simulink model "Rectifier_Buck_Model_rev05_with_Termal_Power_Measurement"  (R2020b)
settings: Solver=VariableStepAuto  StartTime=0.0  StopTime=10  RelTol=1e-3
values from neighbouring files (symbols this model uses):
  L = Vout*(1-D)/(fs*delta_i)    (= 0.001104)    [Parameters.m]
undefined symbols (not defined in the file or in its folder): Acid, Lead
libraries: powerlib x18, electricdrivelib x1, powerlib_meascontrol x1
settings Model: Creator=Alper  LastModifiedBy=faati

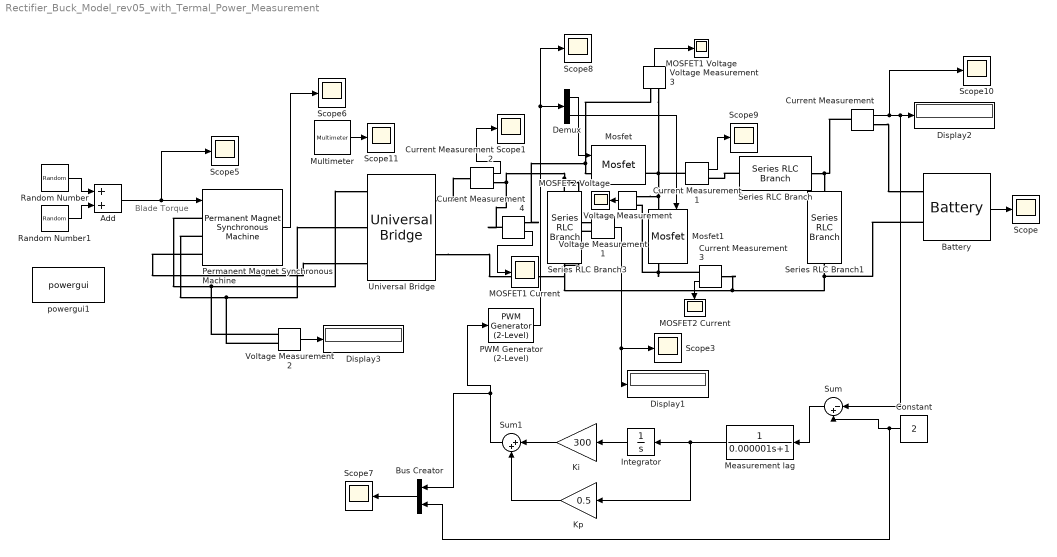
== system Rectifier_Buck_Model_rev05_with_Termal_Power_Measurement ==
  note: Blade Torque
  Add : Sum
  Battery : electricdrivelib/Extra Sources/Battery  BatType=Lead-Acid  ShowTempParam=off  ThermalPreset=no  ShowAgeParam=off  NomV=24  NomQ=5.4  SOC=50  Batt_Tr=30  PresetModel=off  MaxQ=5.625  MinV=18  FullV=26.1316  Dis_rate=1.08  R=0.044444  Normal_OP=1.6755  expZone="[24.4342        0.018]"  current=[6.5 13 32.5]  Units=Time  Tci=20  NomT=20  T2=-30  MaxQ2=4.8  FullV2=7.1  Normal_OP2=5.655  expZone2="[6.58           1]"  Rca=0.6  ti=2000  Dp=0  Neq0=0  Tsim=1e6  Ta1=25  Qeol=5.4*0.9  Reol=0.013333*1.2  Char_age=[2.3478, 3]  Dis_age=[2.3478, 10]  N1=1500  N2=10500  N3=1000  N4=1400  Ta2=45  N5=950
  Bus Creator : BusCreator  Inputs=2
  Constant : Constant  Value=2
  Current Measurement{,1..4} (5 alike) : powerlib/Measurements/Current Measurement  PhasorSimulation=off  OutputType=Complex  PSBequivalent=0
  Demux : Demux  Outputs=2
  Display1 : Display
  Display2 : Display
  Display3 : Display
  Integrator : Integrator
  Ki : Gain  Gain=300
  Kp : Gain  Gain=0.5
  MOSFET1 Current : Scope
  MOSFET1 Voltage : Scope
  MOSFET2 Current : Scope
  MOSFET2 Voltage : Scope
  Measurement lag : TransferFcn  Denominator=[0.000001 1]
  Mosfet : powerlib/Power Electronics/Mosfet  Ron=0.1  Lon=0  Rd=0.01  Vfd=0  IC=0  Rs=1e5  Cs=inf  Measurements=on
  Mosfet1 : powerlib/Power Electronics/Mosfet  Ron=0.1  Lon=0  Rd=0.01  Vfd=0  IC=0  Rs=1e5  Cs=inf  Measurements=on
  Multimeter : powerlib/Measurements/Multimeter  PhasorSimulation=off  OutputType=Complex  sel=[1 2 3 4 5 6]  L=6  Gain=[1 1 1 1 1 1]  yselected={'Isw1: Universal Bridge','Isw2: Universal Bridge','Isw3: Universal Bridge','Isw4: Universal Bridge','Isw5: Universal Bridge','Isw6: Universal Bridge'};  PSBOutputType=1  PSBequivalent=0  AxesSetting=[0,0.1,-100,100]  Display=1  SavedBlockNames=-11
  PWM Generator (2-Level) : powerlib_meascontrol/Pulse & Signal Generators/PWM Generator (2-Level)  ModulatorType=Single-phase half-bridge (2 pulses)  ModulatorMode=Unsynchronized  Fc=50000  Pc=90  nF=27  MinMax="[ -1  1 ]"  SamplingTechnique=Natural  ModulatingSignals=off  m=0.8  Freq=60  Phase=0  Ts=0  ShowCarrierOutport=off
  Permanent Magnet Synchronous Machine : powerlib/Machines/Permanent Magnet Synchronous Machine  NbPhases=3  FluxDistribution=Sinusoidal  RotorType=Round  MechanicalLoad=Torque Tm  PresetModel=No  ShowDetailedParameters=on  MeasurementBus=off  Resistance=10.58  Inductance=8.5e-3  dqInductances=[8.5e-3,8.5e-3]  La=0.0167  MachineConstant=Voltage Constant (V_peak L-L / krpm)  Flux=0.60646  VoltageCst=110  TorqueCst=0.90969  Flat=120  Mechanical=[0.00027 0.005024 1 0]  PolePairs=4  InitialConditions=[300,0, 0,0]  InitialConditions5ph=[0 0 0 0 0 0]  RefAngle=90 degrees behind phase A axis (modified Park)  IterativeDiscreteModel=Trapezoidal non iterative  TsBlock=-1  TsPowergui=0
  Random Number : RandomNumber  Mean=-1.6  Variance=0.05  SampleTime=1
  Random Number1 : RandomNumber  Variance=0.1  SampleTime=1e-3
  Scope{,1,3,5..11} (10 alike) : Scope
  Series RLC Branch : powerlib/Elements/Series RLC Branch  LConnTagsString=__new0  RConnTagsString=__new0  BranchType=L  Resistance=1  Inductance=2.2e-3  SetiL0=off  InitialCurrent=0  Capacitance=1e-6  Setx0=off  InitialVoltage=0  Measurements=None
  Series RLC Branch1 : powerlib/Elements/Series RLC Branch  LConnTagsString=__new0  RConnTagsString=__new0  BranchType=C  Resistance=1  Inductance=1e-3  SetiL0=off  InitialCurrent=0  Capacitance=100e-6  Setx0=off  InitialVoltage=0  Measurements=None
  Series RLC Branch3 : powerlib/Elements/Series RLC Branch  LConnTagsString=__new0  RConnTagsString=__new0  BranchType=C  Resistance=1  Inductance=1e-3  SetiL0=off  InitialCurrent=0  Capacitance=850e-6  Setx0=off  InitialVoltage=0  Measurements=None
  Sum : Sum  Inputs=|-+  InputSameDT=on  SaturateOnIntegerOverflow=on  OutDataTypeStr=Inherit: Same as first input
  Sum1 : Sum  Inputs=|++  InputSameDT=on  SaturateOnIntegerOverflow=on  OutDataTypeStr=Inherit: Same as first input
  Universal Bridge : powerlib/Power Electronics/Universal Bridge  Arms=3  SnubberResistance=1e5  SnubberCapacitance=inf  Device=Diodes  Ron=1e-3  Lon=0  ForwardVoltages="[  0  0  ]"  ForwardVoltage=1.2  GTOparameters=[ 10e-6 , 20e-6 ]  IGBTparameters=[ 1e-6 , 2e-6 ]  Measurements=Device currents  Measurements_2=None  converterType=Rectifier
  Voltage Measurement{,1..3} (4 alike) : powerlib/Measurements/Voltage Measurement  PhasorSimulation=off  OutputType=Complex  PSBequivalent=0
  powergui1 : powerlib/powergui  Priority=1  SimulationMode=Discrete  SampleTime=1e-6  frequency=60  Iterations=50  frequencyindice=0  Pbase=100e6  ErrMax=1e-4  UnitsV=kV  UnitsW=MW  buscounter=0  FunctionMessages=off  echomessages=off  EnableUseOfTLC=off  CurrentSourceSwitches=off  DisableSnubberDevices=off  DisableRonSwitches=off  DisableVfSwitches=off  DisplayEquations=off  AutomaticDiscreteSolvers=off  SolverType=Tustin/Backward Euler (TBE)  Interpol=off  ExternalGateDelay=off  methode=off  Ts=100  x0status=blocks  SPID=on  SwTol=0  HookPort=off  NonlinearTolerance=0  nMaxIteration=15  ContinueOnMaxIteration=off  RestoreLinks=warning  ResistiveCurrentMeasurement=off  Frange=[0:2:500]  Ylog=off  Xlog=on  ShowGrid=off  save=off  variable=ZData  structure=0  ZoomFFT=off  StartTime=0.0  cycles=1  DisplayStyle=1  fundamental=60  FreqAxis=off  MaxFrequency=1000  frequencyindicesteady=1  RmsSteady=1  display=off
  wires:
  Voltage Measurement1/1 -> Display1/1, Scope3/1
  Current Measurement/1 -> Sum/1, Display2/1, Scope10/1
  Random Number1/1 -> Add/2
  Add/1 -> Scope5/1, Permanent Magnet Synchronous Machine/1
  Random Number/1 -> Add/1
  Voltage Measurement2/1 -> Display3/1
  Permanent Magnet Synchronous Machine/1 -> Scope6/1
  Constant/1 -> Bus Creator/2, Sum/2
  Bus Creator/1 -> Scope7/1
  Current Measurement1/1 -> Scope9/1
  Battery/1 -> Scope/1
  Kp/1 -> Sum1/2
  Integrator/1 -> Ki/1
  Measurement lag/1 -> Integrator/1, Kp/1
  Ki/1 -> Sum1/1
  Sum/1 -> Measurement lag/1
  Sum1/1 -> PWM Generator (2-Level)/1, Bus Creator/1
  Current Measurement2/1 -> Scope1/1
  PWM Generator (2-Level)/1 -> Scope8/1, Demux/1
  Demux/1 -> Mosfet/1
  Demux/2 -> Mosfet1/1
  Voltage Measurement/1 -> MOSFET2 Voltage/1
  Current Measurement3/1 -> MOSFET2 Current/1
  Multimeter/1 -> Scope11/1
  Voltage Measurement3/1 -> MOSFET1 Voltage/1
  Current Measurement4/1 -> MOSFET1 Current/1
  connections:
  Series RLC Branch/RConn1 -- Current Measurement/LConn1 -- Series RLC Branch1/LConn1
  Voltage Measurement1/LConn2 -- Universal Bridge/RConn2 -- Series RLC Branch3/RConn1 -- Battery/LConn2 -- Series RLC Branch1/RConn1 -- Current Measurement3/LConn1
  Current Measurement2/RConn1 -- Current Measurement4/LConn1 -- Series RLC Branch3/LConn1 -- Voltage Measurement1/LConn1
  Permanent Magnet Synchronous Machine/LConn1 -- Voltage Measurement2/LConn1 -- Universal Bridge/LConn1
  Permanent Magnet Synchronous Machine/LConn2 -- Voltage Measurement2/LConn2 -- Universal Bridge/LConn2
  Permanent Magnet Synchronous Machine/LConn3 -- Universal Bridge/LConn3
  Series RLC Branch/LConn1 -- Current Measurement1/RConn1
  Current Measurement/RConn1 -- Battery/LConn1
  Universal Bridge/RConn1 -- Current Measurement2/LConn1
  Current Measurement1/LConn1 -- Voltage Measurement3/LConn2 -- Voltage Measurement/LConn1 -- Mosfet1/LConn1 -- Mosfet/RConn1
  Mosfet1/RConn1 -- Current Measurement3/RConn1 -- Voltage Measurement/LConn2
  Voltage Measurement3/LConn1 -- Current Measurement4/RConn1 -- Mosfet/LConn1
